simulink model "function2"  (R2020b)
settings: Solver=VariableStepAuto  StartTime=0.0  StopTime=10.0  RelTol=1e-3
settings Model: Creator=Aurelie  LastModifiedBy=Aurelie

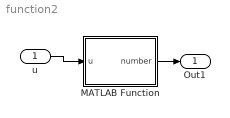
== system function2 ==
  u : Inport
  MATLAB Function : MATLAB Function  TreatAsAtomicUnit=on
  Out1 : Outport
  wires:
  u/1 -> MATLAB Function/1(u)
  MATLAB Function/1(number) -> Out1/1

== matlab function function2/MATLAB Function ==
  data: u input; number output
function number = callrandomNumber(u)
number=randomNumber(u);
end
